simulink model "task2_3"  (R2023a)
settings: Solver=VariableStepAuto  StartTime=0.0  StopTime=10.0  RelTol=1e-8
settings Model: Creator=user  LastModifiedBy=user

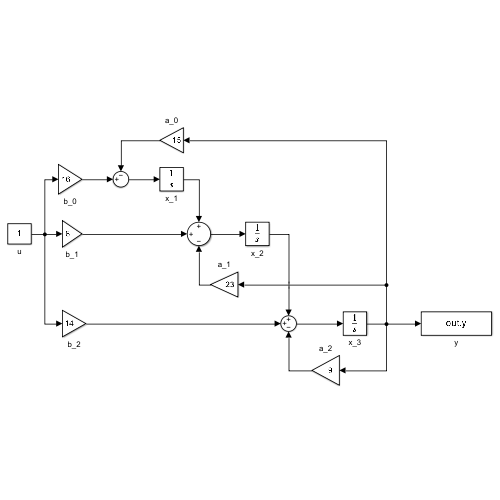
[thumbnail: Simulink's stored preview of the top-level diagram]
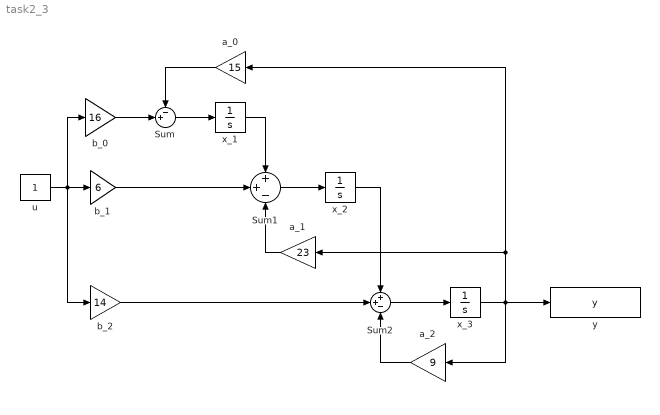
== system task2_3 ==
  Sum : Sum  Inputs=-+|
  Sum1 : Sum  Inputs=++-
  Sum2 : Sum  Inputs=++-
  a_0 : Gain  Gain=15
  a_1 : Gain  Gain=23
  a_2 : Gain  Gain=9
  b_0 : Gain  Gain=16
  b_1 : Gain  Gain=6
  b_2 : Gain  Gain=14
  u : Constant
  x_1 : Integrator
  x_2 : Integrator
  x_3 : Integrator
  y : ToWorkspace  VariableName=y  SaveFormat=Timeseries  SampleTime=-1
  wires:
  u/1 -> b_2/1, b_1/1, b_0/1
  b_0/1 -> Sum/2
  a_0/1 -> Sum/1
  Sum/1 -> x_1/1
  x_1/1 -> Sum1/1
  b_1/1 -> Sum1/2
  a_1/1 -> Sum1/3
  Sum1/1 -> x_2/1
  b_2/1 -> Sum2/2
  a_2/1 -> Sum2/3
  x_2/1 -> Sum2/1
  Sum2/1 -> x_3/1
  x_3/1 -> a_0/1, a_1/1, a_2/1, y/1
